simulink model "Ext_Springs_2SFs"  (R2019a)
settings: Solver=FixedStepDiscrete  StartTime=0  StopTime=10  FixedStep=0.0005  RelTol=1e-3  AbsTol=1e-6
PreLoadFcn:
  | cd Extensions/Simulink/Springs
  | spring_e_class
  | cd ../../..
undefined symbols (not defined in the file): FS_COMP_TABLE_F, FS_COMP_TABLE_R
libraries: Solver_SF x2
settings Model: ExtModeTrigMode=oneshot  ExtModeArmWhenConnect=off  Creator=dhall  LastModifiedBy=msayers
settings SolverCC: AutoScaleAbsTol=off
settings DataIOCC: SaveFormat=Array  ReturnWorkspaceOutputs=off  SignalLoggingName=sigsOut
settings OptimizationCC: BooleanDataType=off  ExpressionDepthLimit=2147483647  LifeSpan=inf
settings DebuggingCC: SaveWithParameterizedLinksMsg=none  UnderspecifiedInitializationDetection=Classic  MergeDetectMultiDrivingBlocksExec=none  SignalResolutionControl=TryResolveAllWithWarning  MultiTaskDSMMsg=warning  MultiTaskCondExecSysMsg=none  FcnCallInpInsideContextMsg=warning  StateNameClashWarn=warning  SFUnexpectedBacktrackingDiag=warning  SFNoUnconditionalDefaultTransitionDiag=warning  ArithmeticOperatorsInVariantConditions=warning
settings HardwareCC: ProdBitPerPointer=32  ProdBitPerSizeT=32  ProdBitPerPtrDiffT=32  ProdLargestAtomicFloat=None  ProdIntDivRoundTo=Undefined  ProdEndianess=Unspecified  ProdWordSize=32  ProdHWDeviceType=32-bit Generic  TargetUnknown=on
settings ModelReferenceCC: PropagateSignalLabelsOutOfModel=off
settings SFSimCC: SimUseLocalCustomCode=off
settings RTWCC: TemplateMakefile=grt_vc.tmf  RTWUseLocalCustomCode=off
settings CodeAppCC: StateflowObjectComments=on
settings GRTTargetCC: TargetFcnLib=ansi_tfl_tmw.mat  TargetLangStandard=C89/C90 (ANSI)  CombineOutputUpdateFcns=off  GRTInterface=on
settings ConfigComp: CovMetricSettings=dw  CovSaveCumulativeToWorkspaceVar=on  CovSaveSingleToWorkspaceVar=on  CovExternalEMLEnable=off  CovSFcnEnable=off

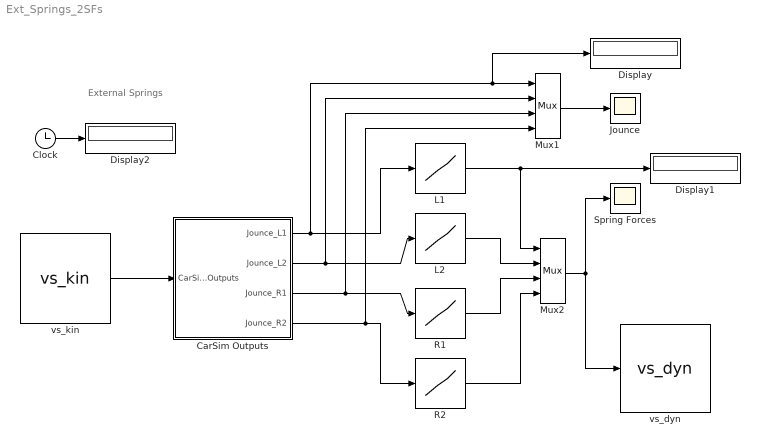
== system Ext_Springs_2SFs ==
  note: External Springs
  CarSim Outputs : Subsystem
  Clock : Clock
  Display : Display
  Display1 : Display
  Display2 : Display
  Jounce : Scope
  L1 : Lookup  InputValues=FS_COMP_TABLE_F(:,1)  Table=FS_COMP_TABLE_F(:,2)  SaturateOnIntegerOverflow=on
  L2 : Lookup  InputValues=FS_COMP_TABLE_R(:,1)  Table=FS_COMP_TABLE_R(:,2)  SaturateOnIntegerOverflow=on
  Mux1 : Mux
  Mux2 : Mux
  R1 : Lookup  InputValues=FS_COMP_TABLE_F(:,1)  Table=FS_COMP_TABLE_F(:,2)  SaturateOnIntegerOverflow=on
  R2 : Lookup  InputValues=FS_COMP_TABLE_R(:,1)  Table=FS_COMP_TABLE_R(:,2)  SaturateOnIntegerOverflow=on
  Spring Forces : Scope
  vs_dyn : Solver_SF/CarSim Multi-Wrappers/vs_dyn  Priority=4  SIMFILE=simfile.sim
  vs_kin : Solver_SF/CarSim Multi-Wrappers/vs_kin  Priority=3  SIMFILE=simfile.sim
  wires:
  Mux1/1 -> Jounce/1
  CarSim Outputs/1(Jounce_L1) -> L1/1, Display/1, Mux1/1
  CarSim Outputs/2(Jounce_L2) -> L2/1, Mux1/2
  CarSim Outputs/3(Jounce_R1) -> R1/1, Mux1/3
  CarSim Outputs/4(Jounce_R2) -> R2/1, Mux1/4
  L1/1 -> Display1/1, Mux2/1
  L2/1 -> Mux2/2
  R1/1 -> Mux2/3
  R2/1 -> Mux2/4
  Clock/1 -> Display2/1
  Mux2/1 -> vs_dyn/1, Spring Forces/1
  vs_kin/1 -> CarSim Outputs/1(CarSim Outputs)

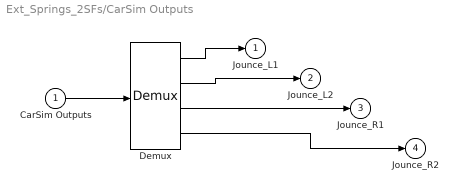
== system Ext_Springs_2SFs/CarSim Outputs ==
  CarSim Outputs : Inport
  Demux : Demux
  Jounce_L1 : Outport  InitialOutput=0
  Jounce_L2 : Outport  Port=2  InitialOutput=0
  Jounce_R1 : Outport  Port=3  InitialOutput=0
  Jounce_R2 : Outport  Port=4  InitialOutput=0
  wires:
  CarSim Outputs/1 -> Demux/1
  Demux/1 -> Jounce_L1/1
  Demux/2 -> Jounce_L2/1
  Demux/3 -> Jounce_R1/1
  Demux/4 -> Jounce_R2/1
